simulink model "sine_wave"  (R2021b)
settings: Solver=VariableStepAuto  StartTime=0.0  StopTime=10.0  RelTol=1e-3
settings Model: Creator=emre-  LastModifiedBy=emre-

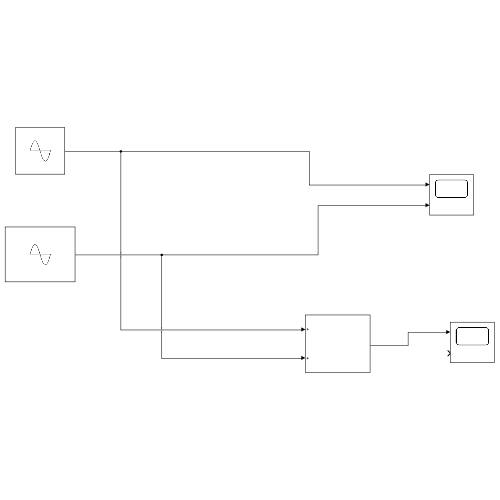
[thumbnail: Simulink's stored preview of the top-level diagram]
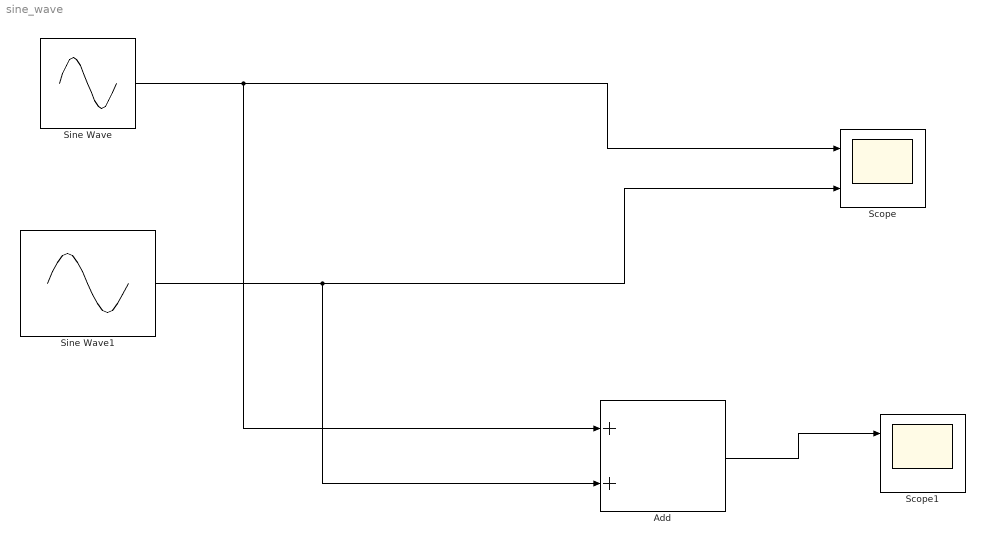
== system sine_wave ==
  Add : Sum
  Scope : Scope  NumInputPorts=2
  Scope1 : Scope  NumInputPorts=2
  Sine Wave : Sin  SampleTime=0
  Sine Wave1 : Sin  Amplitude=2  Frequency=2 * pi  SampleTime=0
  wires:
  Sine Wave/1 -> Add/1, Scope/1
  Sine Wave1/1 -> Add/2, Scope/2
  Add/1 -> Scope1/1
